simulink model "PI1GDL"  (R2018a)
settings: Solver=VariableStepAuto  StartTime=0.0  StopTime=100  RelTol=1e-3
values from neighbouring files (symbols this model uses):
  k = 9.22    [Controlador2GDL.m]    (also in ControladorAlfaroPI1GDL_ControlEstricto.m; ControladorAlfaroPI1GDL_ControlSuave.m; Examen2.m)
  L = 3.17    [Controlador2GDL.m]    (also in ControladorAlfaroPI1GDL_ControlEstricto.m; ControladorAlfaroPI1GDL_ControlSuave.m; Examen2.m)
  T = 34.31    [Controlador2GDL.m]    (also in ControladorAlfaroPI1GDL_ControlEstricto.m; ControladorAlfaroPI1GDL_ControlSuave.m; Examen2.m)
libraries: simulink x1
settings Model: Creator=Rafael  LastModifiedBy=wivill
settings CodeAppCC: StateflowObjectComments=on

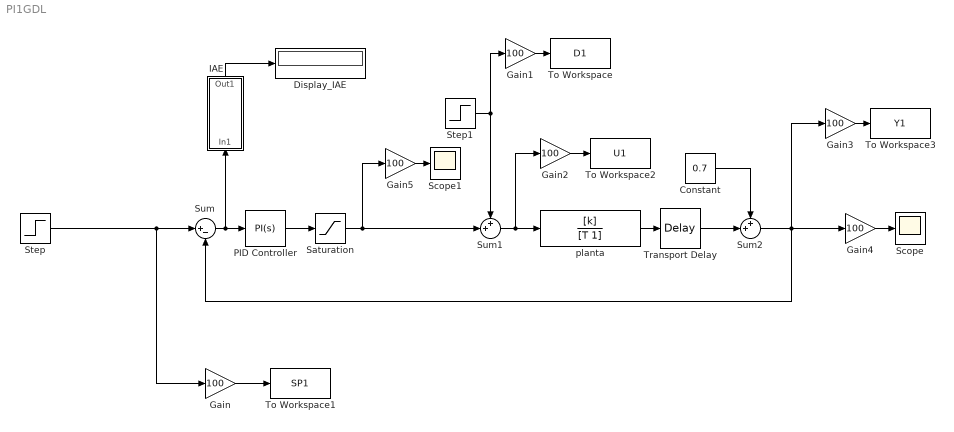
== system PI1GDL ==
  Constant : Constant  Value=0.7
  "Display_IAE " : Display
  Gain{,1..5} (6 alike) : Gain  Gain=100
  IAE : Subsystem
      mask help:
      | IAE performacne index
      |
      | output = int |input| dt
      mask Display:
      | disp('IAE')
      | port_label('input',1,'e')
      | port_label('output',1,'iae')
  PID Controller : simulink/Continuous/PID Controller  Controller=PI  TimeDomain=Continuous-time  SampleTime=-1  IntegratorMethod=Forward Euler  FilterMethod=Forward Euler  Form=Ideal  UseFilter=on  ControllerParametersSource=internal  P=1/(k*(t+(L/T)))  I=1/(T)  D=0  N=100  InitialConditionSource=internal  InitialConditionForIntegrator=0  InitialConditionForFilter=0  ExternalReset=none  LimitOutput=off  UpperSaturationLimit=inf  LowerSaturationLimit=-inf  LinearizeAsGain=on  AntiWindupMode=none  Kb=1  TrackingMode=off  Kt=1  PParamMin=[]  PParamMax=[]  IParamMin=[]  IParamMax=[]  DParamMin=[]  DParamMax=[]  NParamMin=[]  NParamMax=[]  KbParamMin=[]  KbParamMax=[]  KtParamMin=[]  KtParamMax=[]  POutMin=[]  POutMax=[]  IOutMin=[]  IOutMax=[]  DOutMin=[]  DOutMax=[]  NOutMin=[]  NOutMax=[]  KbOutMin=[]  KbOutMax=[]  KtOutMin=[]  KtOutMax=[]  IntegratorOutMin=[]  IntegratorOutMax=[]  FilterOutMin=[]  FilterOutMax=[]  SumOutMin=[]  SumOutMax=[]  SumI1OutMin=[]  SumI1OutMax=[]  SumI2OutMin=[]  SumI2OutMax=[]  SumI3OutMin=[]  SumI3OutMax=[]  SumDOutMin=[]  SumDOutMax=[]  SaturationOutMin=[]  SaturationOutMax=[]  IntegratorContinuousStateAttributes=''  IntegratorStateMustResolveToSignalObject=off  IntegratorRTWStateStorageClass=Auto  FilterContinuousStateAttributes=''  FilterStateMustResolveToSignalObject=off  FilterRTWStateStorageClass=Auto  DifferentiatorICPrevScaledInput=0  DifferentiatorOutMin=[]  DifferentiatorOutMax=[]  InitialConditionSetting=State (most efficient)  FilterDiffOutCoefMin=[]  FilterDiffOutCoefMax=[]  SumDenOutMin=[]  SumDenOutMax=[]  SumNumOutMin=[]  SumNumOutMax=[]  ReciprocalOutMin=[]  ReciprocalOutMax=[]  DivideOutMin=[]  DivideOutMax=[]  TunerSelectOption=Transfer Function Based (PID Tuner App)
  Saturation : Saturate  UpperLimit=1  LowerLimit=-0.1
  Scope : Scope
  Scope1 : Scope
  Step : Step  Time=0  Before=0.7  After=0.8  SampleTime=0
  Step1 : Step  Time=30  After=-0.05  SampleTime=0
  Sum : Sum  Inputs=|+-
  Sum1 : Sum  Inputs=++|
  Sum2 : Sum  Inputs=++|
  To Workspace : ToWorkspace  VariableName=D1  SaveFormat=Timeseries  SampleTime=-1
  To Workspace1 : ToWorkspace  VariableName=SP1  SaveFormat=Timeseries  SampleTime=-1
  To Workspace2 : ToWorkspace  VariableName=U1  SaveFormat=Timeseries  SampleTime=-1
  To Workspace3 : ToWorkspace  VariableName=Y1  SaveFormat=Timeseries  SampleTime=-1
  Transport Delay : TransportDelay  DelayTime=L
  planta : TransferFcn  Numerator=[k]  Denominator=[T 1]  ContinuousStateAttributes='planta'
  wires:
  planta/1 -> Transport Delay/1
  Sum/1 -> IAE/1(In1), PID Controller/1
  Sum1/1 -> Gain2/1, planta/1
  Step1/1 -> Gain1/1, Sum1/1
  Gain/1 -> To Workspace1/1
  Gain1/1 -> To Workspace/1
  Gain2/1 -> To Workspace2/1
  Gain3/1 -> To Workspace3/1
  Gain4/1 -> Scope/1
  IAE/1(Out1) -> "Display_IAE "/1
  Step/1 -> Gain/1, Sum/1
  Constant/1 -> Sum2/1
  Transport Delay/1 -> Sum2/2
  Sum2/1 -> Gain3/1, Sum/2, Gain4/1
  Saturation/1 -> Gain5/1, Sum1/2
  PID Controller/1 -> Saturation/1
  Gain5/1 -> Scope1/1

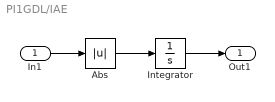
== system PI1GDL/IAE ==
  In1 : Inport
  Abs : Abs
  Integrator : Integrator
  Out1 : Outport
  wires:
  In1/1 -> Abs/1
  Integrator/1 -> Out1/1
  Abs/1 -> Integrator/1
